simulink model "car_speed_tested"  (R2015b)
settings: Solver=FixedStepDiscrete  StartTime=0.0  StopTime=25  RelTol=1e-3
undefined symbols (not defined in the file or in its folder): DiscIntNeverNeededParam
libraries: simulink x5, fuzblock x1
settings Model: Creator=adam  LastModifiedBy=sprinkle
settings DataIOCC: LimitDataPoints=off  SaveFormat=Array
settings HardwareCC: ProdBitPerPointer=32  ProdLargestAtomicFloat=None  ProdIntDivRoundTo=Undefined  ProdEndianess=Unspecified  ProdWordSize=32  ProdHWDeviceType=32-bit Generic
settings GRTTargetCC: GeneratePreprocessorConditionals=Disable all
settings ConfigComp: CovModelRefEnable=Off

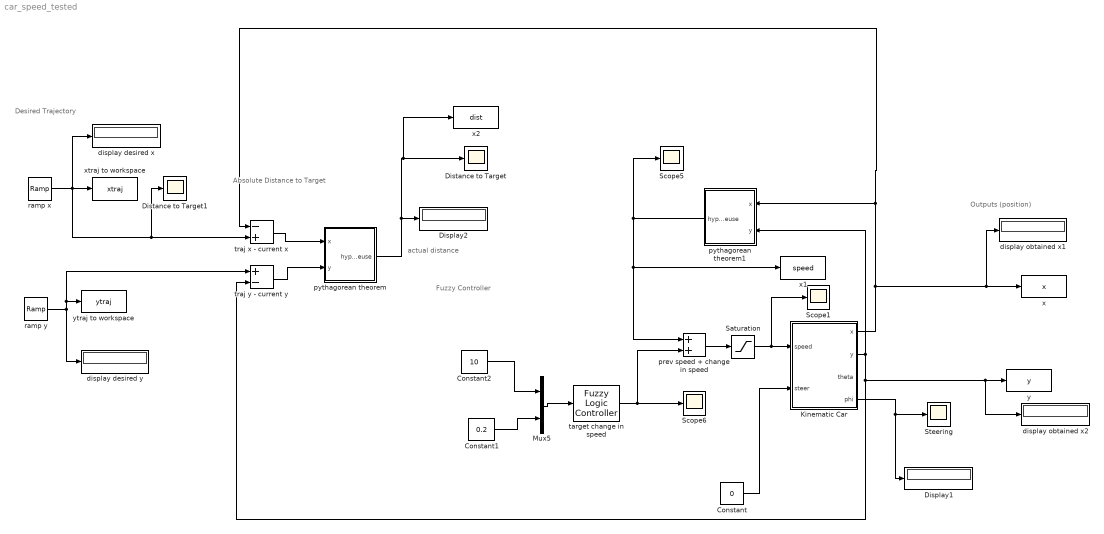
== system car_speed_tested ==
  note: actual distance
  note: Desired Trajectory
  note: Absolute Distance to Target
  note: Fuzzy Controller
  note: Outputs (position)
  Constant : Constant  Value=0
  Constant1 : Constant  Value=0.2
  Constant2 : Constant  Value=10
  Display1 : Display
  Display2 : Display
  Distance to Target : Scope
  Distance to Target1 : Scope
  Kinematic Car : Subsystem
  Mux5 : Mux  Inputs=2
  Saturation : Saturate  UpperLimit=8.9408  LowerLimit=0
  Scope1 : Scope
  Scope5 : Scope
  Scope6 : Scope
  Steering : Scope
  display desired x : Display
  display desired y : Display
  display obtained x1 : Display
  display obtained x2 : Display
  prev speed + change in speed : Sum
  pythagorean theorem : Subsystem
  pythagorean theorem1 : Subsystem
  ramp x : simulink/Sources/Ramp  slope=3  start=0  X0=1
  ramp y : simulink/Sources/Ramp  slope=3  start=0  X0=1
  target change in speed : fuzblock/Fuzzy Logic  Controller  fis='spring2.fis'
  traj x - current x : Sum  Inputs=-+
  traj y - current y : Sum  Inputs=+-
  x : ToWorkspace  VariableName=x  SampleTime=-1
  x1 : ToWorkspace  VariableName=speed  SampleTime=-1
  x2 : ToWorkspace  VariableName=dist  SampleTime=-1
  xtraj to workspace : ToWorkspace  VariableName=xtraj  SampleTime=-1
  y : ToWorkspace  VariableName=y  SampleTime=-1
  ytraj to workspace : ToWorkspace  VariableName=ytraj  SampleTime=-1
  wires:
  Kinematic Car/1(x) -> display obtained x1/1, x/1, traj x - current x/1, pythagorean theorem1/1(x)
  Kinematic Car/2(y) -> y/1, display obtained x2/1, traj y - current y/2, pythagorean theorem1/2(y)
  Mux5/1 -> target change in speed/1
  pythagorean theorem/1(hypoteneuse) -> Display2/1, x2/1, Distance to Target/1
  ramp y/1 -> traj y - current y/1, ytraj to workspace/1, display desired y/1
  pythagorean theorem1/1(hypoteneuse) -> Scope5/1, x1/1, prev speed + change in speed/1
  Kinematic Car/4(phi) -> Display1/1, Steering/1
  target change in speed/1 -> prev speed + change in speed/2, Scope6/1
  prev speed + change in speed/1 -> Saturation/1
  traj x - current x/1 -> pythagorean theorem/1(x)
  traj y - current y/1 -> pythagorean theorem/2(y)
  Constant/1 -> Kinematic Car/2(steer)
  Saturation/1 -> Scope1/1, Kinematic Car/1(speed)
  ramp x/1 -> Distance to Target1/1, traj x - current x/2, xtraj to workspace/1, display desired x/1
  Constant2/1 -> Mux5/1
  Constant1/1 -> Mux5/2

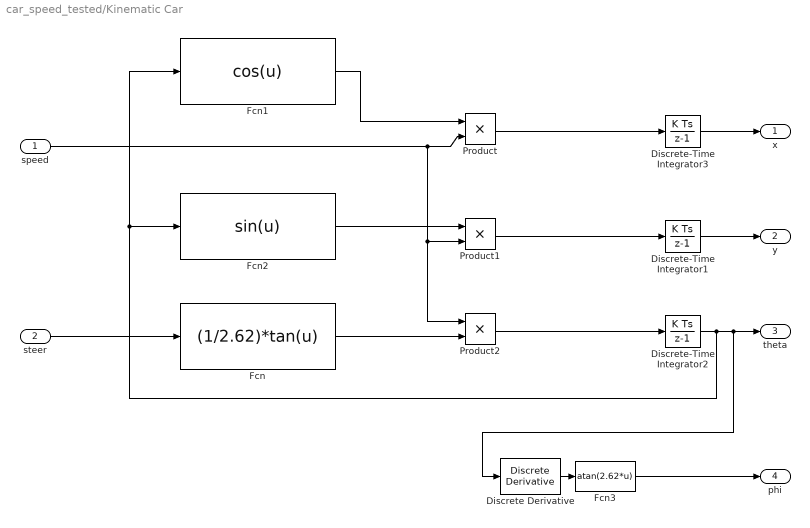
== system car_speed_tested/Kinematic Car ==
  speed : Inport
  steer : Inport  Port=2
  Discrete Derivative : simulink/Discrete/Discrete Derivative  gainval=1.0  ICPrevScaledInput=0.0  InputProcessing=Inherited  OutMin=[]  OutMax=[]  OutDataType=fixdt(1, 16)  OutScaling=2^-10  DoSatur=off
  Discrete-Time Integrator1 : DiscreteIntegrator  InitialConditionSetting=State (most efficient)  ICPrevOutput=DiscIntNeverNeededParam  ICPrevScaledInput=DiscIntNeverNeededParam
  Discrete-Time Integrator2 : DiscreteIntegrator  InitialCondition=atan(pi/4)  InitialConditionSetting=State (most efficient)  ICPrevOutput=DiscIntNeverNeededParam  ICPrevScaledInput=DiscIntNeverNeededParam
  Discrete-Time Integrator3 : DiscreteIntegrator  InitialConditionSetting=State (most efficient)  ICPrevOutput=DiscIntNeverNeededParam  ICPrevScaledInput=DiscIntNeverNeededParam
  Fcn : Fcn  Expr=(1/2.62)*tan(u)
  Fcn1 : Fcn  Expr=cos(u)
  Fcn2 : Fcn  Expr=sin(u)
  Fcn3 : Fcn  Expr=atan(2.62*u)
  Product : Product
  Product1 : Product
  Product2 : Product
  x : Outport
  y : Outport  Port=2
  theta : Outport  Port=3
  phi : Outport  Port=4
  wires:
  Product/1 -> Discrete-Time Integrator3/1
  Product2/1 -> Discrete-Time Integrator2/1
  Fcn1/1 -> Product/1
  Fcn/1 -> Product2/2
  Discrete-Time Integrator2/1 -> Fcn1/1, Fcn2/1, Discrete Derivative/1, theta/1
  Product1/1 -> Discrete-Time Integrator1/1
  Fcn2/1 -> Product1/1
  speed/1 -> Product/2, Product2/1, Product1/2
  steer/1 -> Fcn/1
  Fcn3/1 -> phi/1
  Discrete-Time Integrator3/1 -> x/1
  Discrete-Time Integrator1/1 -> y/1
  Discrete Derivative/1 -> Fcn3/1

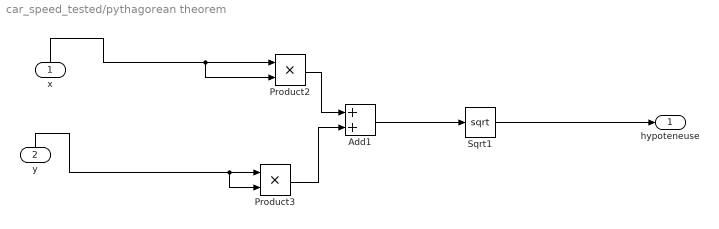
== system car_speed_tested/pythagorean theorem ==
  x : Inport
  y : Inport  Port=2
  Add1 : Sum
  Product2 : Product
  Product3 : Product
  Sqrt1 : Sqrt  SaturateOnIntegerOverflow=on
  hypoteneuse : Outport
  wires:
  Product2/1 -> Add1/1
  Product3/1 -> Add1/2
  Add1/1 -> Sqrt1/1
  Sqrt1/1 -> hypoteneuse/1
  y/1 -> Product3/2, Product3/1
  x/1 -> Product2/2, Product2/1

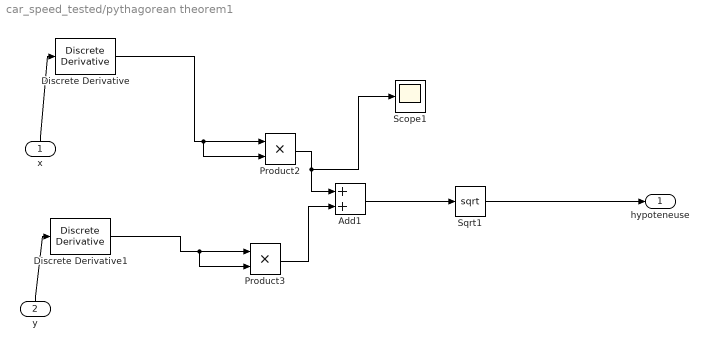
== system car_speed_tested/pythagorean theorem1 ==
  x : Inport
  y : Inport  Port=2
  Add1 : Sum
  Discrete Derivative : simulink/Discrete/Discrete Derivative  gainval=1.0  ICPrevScaledInput=0.0  InputProcessing=Inherited  OutMin=[]  OutMax=[]  OutDataType=fixdt(1, 16)  OutScaling=2^-10  DoSatur=off
  Discrete Derivative1 : simulink/Discrete/Discrete Derivative  gainval=1.0  ICPrevScaledInput=0.0  InputProcessing=Inherited  OutMin=[]  OutMax=[]  OutDataType=fixdt(1, 16)  OutScaling=2^-10  DoSatur=off
  Product2 : Product
  Product3 : Product
  Scope1 : Scope
  Sqrt1 : Sqrt  SaturateOnIntegerOverflow=on
  hypoteneuse : Outport
  wires:
  Product2/1 -> Scope1/1, Add1/1
  Product3/1 -> Add1/2
  Add1/1 -> Sqrt1/1
  Sqrt1/1 -> hypoteneuse/1
  x/1 -> Discrete Derivative/1
  y/1 -> Discrete Derivative1/1
  Discrete Derivative1/1 -> Product3/2, Product3/1
  Discrete Derivative/1 -> Product2/2, Product2/1
